simulink model "Robot"  (R2022b)
settings: Solver=FixedStepDiscrete  StartTime=0.0  StopTime=30  FixedStep=0.001  RelTol=1e-3
InitFcn:
  | load("BusConfig.mat");
undefined symbols (not defined in the file or in its folder): DiscIntNeverNeededParam
libraries: slrealtimeethercatlib x119, simulink x20
(part 4 of 7)

== system Robot/Motor4 Torque Control Init Frame/SDO Set 0x6040:6 Frame ==
  FinishIndex : Inport
  Enable : EnablePort
  Bitwise Operator : simulink/Logic and Bit Operations/Bitwise Operator  logicop=AND  UseBitMask=on  BitMask=bin2dec('0000000000000001')  BitMaskRealWorld=Stored Integer
  Clock : Clock
  Constant : Constant  Value=6  OutDataTypeStr=uint16
  Constant1 : Constant  OutDataTypeStr=int32
  Constant2 : Constant  Value=0  OutDataTypeStr=int32
  Constant4 : Constant  Value=0  OutDataTypeStr=double
  Constant5 : Constant
  Constant6 : Constant  OutDataTypeStr=int32
  Constant7 : Constant
  Constant8 : Constant  Value=0b0000000000000001  OutDataTypeStr=uint16
  Display{1..6} (6 alike) : Display
  EtherCAT Async SDO Download : slrealtimeethercatlib/EtherCAT Async SDO Download  index=0x6040  subIndex=0  sig_type=uint16  sig_dim=1  device_id=0  slave_name=Drive 4 (Elmo Drive )  sample_time=-1  slave_addr=1004  selected_slave=Term 1 (EK1100)  timeout=3000  slave_found=1  complete=0
  EtherCAT PDO Receive1 : slrealtimeethercatlib/EtherCAT PDO Receive  Priority=2  sig_name=Drive 4 (Elmo Drive ).Inputs.Status word  sig_offset=39136  sig_type=uint16  type_size=16  sig_dim=1  device_id=0  sample_time=0.001
  If Action Subsystem1 : Subsystem  TreatAsAtomicUnit=on
  If Action Subsystem2 : Subsystem  TreatAsAtomicUnit=on
  If Action Subsystem3 : Subsystem  TreatAsAtomicUnit=on
  If Action Subsystem5 : Subsystem  TreatAsAtomicUnit=on
  If Action Subsystem6 : Subsystem  TreatAsAtomicUnit=on
  If Action Subsystem7 : Subsystem  TreatAsAtomicUnit=on
  If1 : If  IfExpression=(u1 == 4663)
  If2 : If  IfExpression=(u1 == 2)
  If3 : If  NumInputs=2  IfExpression=(u1 == u2)
  If4 : If  IfExpression=(u1 >= 0.1)
  Merge1 : Merge
  Merge2 : Merge
  TaskFinished : Outport
  wires:
  Constant2/1 -> If Action Subsystem1/1(In1)
  Constant/1 -> EtherCAT Async SDO Download/1
  If1/1 -> If Action Subsystem7/Action
  Constant4/1 -> If Action Subsystem6/1(In1)
  If4/1 -> If Action Subsystem1/Action
  If Action Subsystem1/1(Out1) -> Merge2/1
  If2/2 -> If Action Subsystem6/Action
  Bitwise Operator/1 -> If3/1
  FinishIndex/1 -> If Action Subsystem5/1(In1)
  EtherCAT Async SDO Download/2 -> Display2/1
  EtherCAT Async SDO Download/1 -> If2/1, Display1/1
  If2/1 -> If Action Subsystem5/Action
  If4/2 -> If Action Subsystem2/Action
  Constant5/1 -> If Action Subsystem7/1(In1)
  If Action Subsystem2/1(Out1) -> Merge2/2
  Constant7/1 -> If Action Subsystem3/1(In1)
  If Action Subsystem3/1(Out1) -> Display6/1, If4/1
  If Action Subsystem5/1(Out1) -> Merge1/1
  Constant6/1 -> If Action Subsystem2/1(In1)
  If Action Subsystem6/1(Out1) -> Merge1/2
  Constant1/1 -> EtherCAT Async SDO Download/2
  If3/1 -> If Action Subsystem3/Action
  If Action Subsystem7/1(Out1) -> Display5/1
  Constant8/1 -> If3/2
  EtherCAT PDO Receive1/1 -> Display3/1, Bitwise Operator/1
  Clock/1 -> Display4/1
  Merge1/1 -> TaskFinished/1

== system Robot/Motor4 Torque Control Init Frame/SDO Set 0x6040:7 Frame ==
  FinishIndex : Inport
  Enable : EnablePort
  Bitwise Operator : simulink/Logic and Bit Operations/Bitwise Operator  logicop=AND  UseBitMask=on  BitMask=bin2dec('0000000000000011')  BitMaskRealWorld=Stored Integer
  Clock : Clock
  Constant : Constant  Value=7  OutDataTypeStr=uint16
  Constant1 : Constant  OutDataTypeStr=int32
  Constant2 : Constant  Value=0  OutDataTypeStr=int32
  Constant4 : Constant  Value=0  OutDataTypeStr=double
  Constant5 : Constant
  Constant6 : Constant  OutDataTypeStr=int32
  Constant7 : Constant
  Constant8 : Constant  Value=0b0000000000000011  OutDataTypeStr=uint16
  Display{1..6} (6 alike) : Display
  EtherCAT Async SDO Download : slrealtimeethercatlib/EtherCAT Async SDO Download  index=0x6040  subIndex=0  sig_type=uint16  sig_dim=1  device_id=0  slave_name=Drive 4 (Elmo Drive )  sample_time=-1  slave_addr=1004  selected_slave=Term 1 (EK1100)  timeout=2000  slave_found=1  complete=0
  EtherCAT PDO Receive1 : slrealtimeethercatlib/EtherCAT PDO Receive  Priority=2  sig_name=Drive 4 (Elmo Drive ).Inputs.Status word  sig_offset=39136  sig_type=uint16  type_size=16  sig_dim=1  device_id=0  sample_time=0.001
  If Action Subsystem1 : Subsystem  TreatAsAtomicUnit=on
  If Action Subsystem2 : Subsystem  TreatAsAtomicUnit=on
  If Action Subsystem3 : Subsystem  TreatAsAtomicUnit=on
  If Action Subsystem5 : Subsystem  TreatAsAtomicUnit=on
  If Action Subsystem6 : Subsystem  TreatAsAtomicUnit=on
  If Action Subsystem7 : Subsystem  TreatAsAtomicUnit=on
  If1 : If  IfExpression=(u1 == 4663)
  If2 : If  IfExpression=(u1 == 2)
  If3 : If  NumInputs=2  IfExpression=(u1 == u2)
  If4 : If  IfExpression=(u1 >= 0.1)
  Merge1 : Merge
  Merge2 : Merge
  TaskFinished : Outport
  wires:
  EtherCAT PDO Receive1/1 -> Display3/1, Bitwise Operator/1
  Constant1/1 -> EtherCAT Async SDO Download/2
  Constant/1 -> EtherCAT Async SDO Download/1
  If Action Subsystem1/1(Out1) -> Merge2/1
  Constant7/1 -> If Action Subsystem3/1(In1)
  EtherCAT Async SDO Download/2 -> Display2/1
  Constant4/1 -> If Action Subsystem6/1(In1)
  FinishIndex/1 -> If Action Subsystem5/1(In1)
  If Action Subsystem6/1(Out1) -> Merge1/2
  Constant2/1 -> If Action Subsystem1/1(In1)
  If Action Subsystem5/1(Out1) -> Merge1/1
  Constant5/1 -> If Action Subsystem7/1(In1)
  If4/2 -> If Action Subsystem2/Action
  If2/1 -> If Action Subsystem5/Action
  If Action Subsystem7/1(Out1) -> Display5/1
  Merge1/1 -> TaskFinished/1
  Constant6/1 -> If Action Subsystem2/1(In1)
  Bitwise Operator/1 -> If3/1
  If Action Subsystem3/1(Out1) -> Display6/1, If4/1
  If1/1 -> If Action Subsystem7/Action
  If4/1 -> If Action Subsystem1/Action
  Clock/1 -> Display4/1
  If3/1 -> If Action Subsystem3/Action
  If Action Subsystem2/1(Out1) -> Merge2/2
  Constant8/1 -> If3/2
  If2/2 -> If Action Subsystem6/Action
  EtherCAT Async SDO Download/1 -> If2/1, Display1/1

== system Robot/Motor4 Torque Control Init Frame/SDO Set 0x6060:10 Frame ==
  FinishIndex : Inport
  Enable : EnablePort
  Clock : Clock
  Constant : Constant  Value=10  OutDataTypeStr=int8
  Constant1 : Constant  OutDataTypeStr=int32
  Constant4 : Constant  Value=0  OutDataTypeStr=double
  Constant5 : Constant
  Display{1..2,4..5} (4 alike) : Display
  EtherCAT Async SDO Download : slrealtimeethercatlib/EtherCAT Async SDO Download  index=0x6060  subIndex=0  sig_type=int8  sig_dim=1  device_id=0  slave_name=Drive 4 (Elmo Drive )  sample_time=-1  slave_addr=1004  selected_slave=Term 1 (EK1100)  timeout=2000  slave_found=1  complete=0
  If Action Subsystem5 : Subsystem  TreatAsAtomicUnit=on
  If Action Subsystem6 : Subsystem  TreatAsAtomicUnit=on
  If Action Subsystem7 : Subsystem  TreatAsAtomicUnit=on
  If1 : If  IfExpression=(u1 == 4663)
  If2 : If  IfExpression=(u1 == 2)
  Merge1 : Merge
  TaskFinished : Outport
  wires:
  EtherCAT Async SDO Download/2 -> Display2/1
  If Action Subsystem7/1(Out1) -> Display5/1
  If Action Subsystem6/1(Out1) -> Merge1/2
  If2/1 -> If Action Subsystem5/Action
  If2/2 -> If Action Subsystem6/Action
  Constant/1 -> EtherCAT Async SDO Download/1
  If1/1 -> If Action Subsystem7/Action
  Merge1/1 -> TaskFinished/1
  If Action Subsystem5/1(Out1) -> Merge1/1
  Constant5/1 -> If Action Subsystem7/1(In1)
  Clock/1 -> Display4/1
  Constant1/1 -> EtherCAT Async SDO Download/2
  Constant4/1 -> If Action Subsystem6/1(In1)
  FinishIndex/1 -> If Action Subsystem5/1(In1)
  EtherCAT Async SDO Download/1 -> If2/1, Display1/1

== system Robot/Motor4 Torque Control Init Frame/SDO Set 0x6060:6 Frame ==
  FinishIndex : Inport
  Enable : EnablePort
  Clock : Clock
  Constant : Constant  Value=6  OutDataTypeStr=int8
  Constant1 : Constant  OutDataTypeStr=int32
  Constant4 : Constant  Value=0  OutDataTypeStr=double
  Constant5 : Constant
  Display{1..2,4..5} (4 alike) : Display
  EtherCAT Async SDO Download : slrealtimeethercatlib/EtherCAT Async SDO Download  index=0x6060  subIndex=0  sig_type=int8  sig_dim=1  device_id=0  slave_name=Drive 4 (Elmo Drive )  sample_time=-1  slave_addr=1004  selected_slave=Term 1 (EK1100)  timeout=2000  slave_found=1  complete=0
  If Action Subsystem5 : Subsystem  TreatAsAtomicUnit=on
  If Action Subsystem6 : Subsystem  TreatAsAtomicUnit=on
  If Action Subsystem7 : Subsystem  TreatAsAtomicUnit=on
  If1 : If  IfExpression=(u1 == 4663)
  If2 : If  IfExpression=(u1 == 2)
  Merge1 : Merge
  TaskFinished : Outport
  wires:
  FinishIndex/1 -> If Action Subsystem5/1(In1)
  If2/1 -> If Action Subsystem5/Action
  If Action Subsystem5/1(Out1) -> Merge1/1
  If Action Subsystem6/1(Out1) -> Merge1/2
  EtherCAT Async SDO Download/2 -> Display2/1
  If2/2 -> If Action Subsystem6/Action
  Constant1/1 -> EtherCAT Async SDO Download/2
  Merge1/1 -> TaskFinished/1
  If Action Subsystem7/1(Out1) -> Display5/1
  Clock/1 -> Display4/1
  EtherCAT Async SDO Download/1 -> If2/1, Display1/1
  Constant4/1 -> If Action Subsystem6/1(In1)
  Constant5/1 -> If Action Subsystem7/1(In1)
  If1/1 -> If Action Subsystem7/Action
  Constant/1 -> EtherCAT Async SDO Download/1

== system Robot/Motor4 Torque Control Init Frame/SDO Set 0x6080:-1 Frame ==
  FinishIndex : Inport
  Enable : EnablePort
  Clock : Clock
  Constant : Constant  Value=(2^31)-1  OutDataTypeStr=int32
  Constant1 : Constant  OutDataTypeStr=int32
  Constant4 : Constant  Value=0  OutDataTypeStr=double
  Constant5 : Constant
  Display{1..2,4..5} (4 alike) : Display
  EtherCAT Async SDO Download : slrealtimeethercatlib/EtherCAT Async SDO Download  index=0x6080  subIndex=0  sig_type=int32  sig_dim=1  device_id=0  slave_name=Drive 4 (Elmo Drive )  sample_time=-1  slave_addr=1004  selected_slave=Term 1 (EK1100)  timeout=3000  slave_found=1  complete=0
  If Action Subsystem5 : Subsystem  TreatAsAtomicUnit=on
  If Action Subsystem6 : Subsystem  TreatAsAtomicUnit=on
  If Action Subsystem7 : Subsystem  TreatAsAtomicUnit=on
  If1 : If  IfExpression=(u1 == 4663)
  If2 : If  IfExpression=(u1 == 2)
  Merge1 : Merge
  TaskFinished : Outport
  wires:
  Merge1/1 -> TaskFinished/1
  EtherCAT Async SDO Download/1 -> If2/1, Display1/1
  EtherCAT Async SDO Download/2 -> Display2/1
  Constant1/1 -> EtherCAT Async SDO Download/2
  FinishIndex/1 -> If Action Subsystem5/1(In1)
  If2/2 -> If Action Subsystem6/Action
  If2/1 -> If Action Subsystem5/Action
  Constant4/1 -> If Action Subsystem6/1(In1)
  Constant/1 -> EtherCAT Async SDO Download/1
  Constant5/1 -> If Action Subsystem7/1(In1)
  Clock/1 -> Display4/1
  If1/1 -> If Action Subsystem7/Action
  If Action Subsystem7/1(Out1) -> Display5/1
  If Action Subsystem6/1(Out1) -> Merge1/2
  If Action Subsystem5/1(Out1) -> Merge1/1

== system Robot/Motor4 Torque Control Init Frame/SDO Set 0x6098:35 Frame ==
  FinishIndex : Inport
  Enable : EnablePort
  Clock : Clock
  Constant : Constant  Value=35  OutDataTypeStr=int8
  Constant1 : Constant  OutDataTypeStr=int32
  Constant4 : Constant  Value=0  OutDataTypeStr=double
  Constant5 : Constant
  Display{1..2,4..5} (4 alike) : Display
  EtherCAT Async SDO Download : slrealtimeethercatlib/EtherCAT Async SDO Download  index=0x6098  subIndex=0  sig_type=int8  sig_dim=1  device_id=0  slave_name=Drive 4 (Elmo Drive )  sample_time=-1  slave_addr=1004  selected_slave=Term 1 (EK1100)  timeout=2000  slave_found=1  complete=0
  If Action Subsystem5 : Subsystem  TreatAsAtomicUnit=on
  If Action Subsystem6 : Subsystem  TreatAsAtomicUnit=on
  If Action Subsystem7 : Subsystem  TreatAsAtomicUnit=on
  If1 : If  IfExpression=(u1 == 4663)
  If2 : If  IfExpression=(u1 == 2)
  Merge1 : Merge
  TaskFinished : Outport
  wires:
  EtherCAT Async SDO Download/2 -> Display2/1
  EtherCAT Async SDO Download/1 -> If2/1, Display1/1
  Constant1/1 -> EtherCAT Async SDO Download/2
  FinishIndex/1 -> If Action Subsystem5/1(In1)
  Constant4/1 -> If Action Subsystem6/1(In1)
  If Action Subsystem5/1(Out1) -> Merge1/1
  Constant5/1 -> If Action Subsystem7/1(In1)
  Merge1/1 -> TaskFinished/1
  If2/1 -> If Action Subsystem5/Action
  If Action Subsystem7/1(Out1) -> Display5/1
  Constant/1 -> EtherCAT Async SDO Download/1
  If2/2 -> If Action Subsystem6/Action
  If Action Subsystem6/1(Out1) -> Merge1/2
  If1/1 -> If Action Subsystem7/Action
  Clock/1 -> Display4/1

== system Robot/Motor4 Torque Control Init Frame/Set MasterState to OP Frame ==
  FinishIndex : Inport
  Enable : EnablePort
  Clock : Clock
  Constant1 : Constant  OutDataTypeStr=boolean
  Constant2 : Constant  Value=8  OutDataTypeStr=int32
  Constant4 : Constant  Value=0  OutDataTypeStr=double
  Constant5 : Constant
  Display{1..2,4..5} (4 alike) : Display
  If Action Subsystem5 : Subsystem  TreatAsAtomicUnit=on
  If Action Subsystem6 : Subsystem  TreatAsAtomicUnit=on
  If Action Subsystem7 : Subsystem  TreatAsAtomicUnit=on
  If1 : If  IfExpression=(u1 == 8)
  If2 : If  IfExpression=(u1 > 0.1)
  Merge1 : Merge
  Set Device State : slrealtimeethercatlib/Set Device State  device_id=0  slave_name=Drive 4 (Elmo Drive )  sample_time=-1  slave_addr=1004  selected_slave=Term 1 (EK1100)  slave_found=1
  TaskFinished : Outport
  wires:
  Set Device State/1 -> If1/1, Display1/1
  Merge1/1 -> TaskFinished/1
  Constant1/1 -> Set Device State/2
  Constant4/1 -> If Action Subsystem6/1(In1)
  If1/1 -> If Action Subsystem7/Action
  FinishIndex/1 -> If Action Subsystem5/1(In1)
  Clock/1 -> Display4/1
  Set Device State/2 -> Display2/1
  If Action Subsystem5/1(Out1) -> Merge1/1
  If2/2 -> If Action Subsystem6/Action
  If2/1 -> If Action Subsystem5/Action
  If Action Subsystem7/1(Out1) -> If2/1, Display5/1
  If Action Subsystem6/1(Out1) -> Merge1/2
  Constant2/1 -> Set Device State/1
  Constant5/1 -> If Action Subsystem7/1(In1)

== system Robot/Motor4 Torque Control Init Frame/Set MasterState to SafeOP Frame ==
  FinishIndex : Inport
  Enable : EnablePort
  Clock : Clock
  Constant1 : Constant  OutDataTypeStr=boolean
  Constant2 : Constant  Value=4  OutDataTypeStr=int32
  Constant4 : Constant  Value=0  OutDataTypeStr=double
  Constant5 : Constant
  Display{1..2,4..5} (4 alike) : Display
  If Action Subsystem5 : Subsystem  TreatAsAtomicUnit=on
  If Action Subsystem6 : Subsystem  TreatAsAtomicUnit=on
  If Action Subsystem7 : Subsystem  TreatAsAtomicUnit=on
  If1 : If  IfExpression=(u1 == 4)
  If2 : If  IfExpression=(u1 > 0.1)
  Merge1 : Merge
  Set Device State : slrealtimeethercatlib/Set Device State  device_id=0  slave_name=Drive 4 (Elmo Drive )  sample_time=-1  slave_addr=1004  selected_slave=Term 1 (EK1100)  slave_found=1
  TaskFinished : Outport
  wires:
  Merge1/1 -> TaskFinished/1
  Set Device State/1 -> If1/1, Display1/1
  Constant1/1 -> Set Device State/2
  Constant2/1 -> Set Device State/1
  If Action Subsystem7/1(Out1) -> If2/1, Display5/1
  Constant5/1 -> If Action Subsystem7/1(In1)
  Clock/1 -> Display4/1
  If1/1 -> If Action Subsystem7/Action
  If2/1 -> If Action Subsystem5/Action
  If2/2 -> If Action Subsystem6/Action
  Set Device State/2 -> Display2/1
  If Action Subsystem6/1(Out1) -> Merge1/2
  Constant4/1 -> If Action Subsystem6/1(In1)
  FinishIndex/1 -> If Action Subsystem5/1(In1)
  If Action Subsystem5/1(Out1) -> Merge1/1

== system Robot/Motor4 Torque Control Init Frame/State_10_Enable ==
  State : Inport
  Subsystem : Subsystem
  Switch Case : SwitchCase  CaseConditions={TaskIndex}
  Enable : Outport
  FinishIndex : Outport  Port=2
  wires:
  Switch Case/2 -> Subsystem/2(Case Default)
  Switch Case/1 -> Subsystem/1(Case)
  Subsystem/2(FinishIndex) -> FinishIndex/1
  Subsystem/1(Enable) -> Enable/1
  State/1 -> Switch Case/1

== system Robot/Motor4 Torque Control Init Frame/State_11_Enable ==
  State : Inport
  Subsystem : Subsystem
  Switch Case : SwitchCase  CaseConditions={TaskIndex}
  Enable : Outport
  FinishIndex : Outport  Port=2
  wires:
  Switch Case/2 -> Subsystem/2(Case Default)
  Switch Case/1 -> Subsystem/1(Case)
  Subsystem/2(FinishIndex) -> FinishIndex/1
  Subsystem/1(Enable) -> Enable/1
  State/1 -> Switch Case/1

== system Robot/Motor4 Torque Control Init Frame/State_12_Enable ==
  State : Inport
  Subsystem : Subsystem
  Switch Case : SwitchCase  CaseConditions={TaskIndex}
  Enable : Outport
  FinishIndex : Outport  Port=2
  wires:
  Switch Case/2 -> Subsystem/2(Case Default)
  Switch Case/1 -> Subsystem/1(Case)
  Subsystem/2(FinishIndex) -> FinishIndex/1
  Subsystem/1(Enable) -> Enable/1
  State/1 -> Switch Case/1

== system Robot/Motor4 Torque Control Init Frame/State_13_Enable ==
  State : Inport
  Subsystem : Subsystem
  Switch Case : SwitchCase  CaseConditions={TaskIndex}
  Enable : Outport
  FinishIndex : Outport  Port=2
  wires:
  Switch Case/2 -> Subsystem/2(Case Default)
  Switch Case/1 -> Subsystem/1(Case)
  Subsystem/2(FinishIndex) -> FinishIndex/1
  Subsystem/1(Enable) -> Enable/1
  State/1 -> Switch Case/1

== system Robot/Motor4 Torque Control Init Frame/State_1_Enable ==
  State : Inport
  Subsystem : Subsystem
  Switch Case : SwitchCase  CaseConditions={TaskIndex}
  Enable : Outport
  FinishIndex : Outport  Port=2
  wires:
  Switch Case/2 -> Subsystem/2(Case Default)
  Switch Case/1 -> Subsystem/1(Case)
  Subsystem/2(FinishIndex) -> FinishIndex/1
  Subsystem/1(Enable) -> Enable/1
  State/1 -> Switch Case/1

== system Robot/Motor4 Torque Control Init Frame/State_2_Enable ==
  State : Inport
  Subsystem : Subsystem
  Switch Case : SwitchCase  CaseConditions={TaskIndex}
  Enable : Outport
  FinishIndex : Outport  Port=2
  wires:
  Switch Case/2 -> Subsystem/2(Case Default)
  Switch Case/1 -> Subsystem/1(Case)
  Subsystem/2(FinishIndex) -> FinishIndex/1
  Subsystem/1(Enable) -> Enable/1
  State/1 -> Switch Case/1

== system Robot/Motor4 Torque Control Init Frame/State_3_Enable ==
  State : Inport
  Subsystem : Subsystem
  Switch Case : SwitchCase  CaseConditions={TaskIndex}
  Enable : Outport
  FinishIndex : Outport  Port=2
  wires:
  Switch Case/2 -> Subsystem/2(Case Default)
  Switch Case/1 -> Subsystem/1(Case)
  Subsystem/2(FinishIndex) -> FinishIndex/1
  Subsystem/1(Enable) -> Enable/1
  State/1 -> Switch Case/1

== system Robot/Motor4 Torque Control Init Frame/State_4_Enable ==
  State : Inport
  Subsystem : Subsystem
  Switch Case : SwitchCase  CaseConditions={TaskIndex}
  Enable : Outport
  FinishIndex : Outport  Port=2
  wires:
  Switch Case/2 -> Subsystem/2(Case Default)
  Switch Case/1 -> Subsystem/1(Case)
  Subsystem/2(FinishIndex) -> FinishIndex/1
  Subsystem/1(Enable) -> Enable/1
  State/1 -> Switch Case/1

== system Robot/Motor4 Torque Control Init Frame/State_5_Enable ==
  State : Inport
  Subsystem : Subsystem
  Switch Case : SwitchCase  CaseConditions={TaskIndex}
  Enable : Outport
  FinishIndex : Outport  Port=2
  wires:
  Switch Case/2 -> Subsystem/2(Case Default)
  Switch Case/1 -> Subsystem/1(Case)
  Subsystem/2(FinishIndex) -> FinishIndex/1
  Subsystem/1(Enable) -> Enable/1
  State/1 -> Switch Case/1

== system Robot/Motor4 Torque Control Init Frame/State_6_Enable ==
  State : Inport
  Subsystem : Subsystem
  Switch Case : SwitchCase  CaseConditions={TaskIndex}
  Enable : Outport
  FinishIndex : Outport  Port=2
  wires:
  Switch Case/2 -> Subsystem/2(Case Default)
  Switch Case/1 -> Subsystem/1(Case)
  Subsystem/2(FinishIndex) -> FinishIndex/1
  Subsystem/1(Enable) -> Enable/1
  State/1 -> Switch Case/1

== system Robot/Motor4 Torque Control Init Frame/State_7_Enable ==
  State : Inport
  Subsystem : Subsystem
  Switch Case : SwitchCase  CaseConditions={TaskIndex}
  Enable : Outport
  FinishIndex : Outport  Port=2
  wires:
  Switch Case/2 -> Subsystem/2(Case Default)
  Switch Case/1 -> Subsystem/1(Case)
  Subsystem/2(FinishIndex) -> FinishIndex/1
  Subsystem/1(Enable) -> Enable/1
  State/1 -> Switch Case/1

== system Robot/Motor4 Torque Control Init Frame/State_8_Enable ==
  State : Inport
  Subsystem : Subsystem
  Switch Case : SwitchCase  CaseConditions={TaskIndex}
  Enable : Outport
  FinishIndex : Outport  Port=2
  wires:
  Switch Case/2 -> Subsystem/2(Case Default)
  Switch Case/1 -> Subsystem/1(Case)
  Subsystem/2(FinishIndex) -> FinishIndex/1
  Subsystem/1(Enable) -> Enable/1
  State/1 -> Switch Case/1

== system Robot/Motor4 Torque Control Init Frame/State_9_Enable ==
  State : Inport
  Subsystem : Subsystem
  Switch Case : SwitchCase  CaseConditions={TaskIndex}
  Enable : Outport
  FinishIndex : Outport  Port=2
  wires:
  Switch Case/2 -> Subsystem/2(Case Default)
  Switch Case/1 -> Subsystem/1(Case)
  Subsystem/2(FinishIndex) -> FinishIndex/1
  Subsystem/1(Enable) -> Enable/1
  State/1 -> Switch Case/1

== system Robot/State_1_Enable/Subsystem ==
  Case : Inport
  Case Default : Inport  Port=2
  Constant : Constant
  Constant1 : Constant  Value=0
  Constant2 : Constant  Value=TaskIndex
  Merge : Merge
  Switch Case Action Subsystem : Subsystem  TreatAsAtomicUnit=on
  Switch Case Action Subsystem1 : Subsystem  TreatAsAtomicUnit=on
  Enable : Outport
  FinishIndex : Outport  Port=2
  wires:
  Constant/1 -> Switch Case Action Subsystem/1(In1)
  Case/1 -> Switch Case Action Subsystem/Action
  Switch Case Action Subsystem/1(Out1) -> Merge/1
  Merge/1 -> Enable/1
  Case Default/1 -> Switch Case Action Subsystem1/Action
  Constant1/1 -> Switch Case Action Subsystem1/1(In1)
  Switch Case Action Subsystem1/1(Default) -> Merge/2
  Constant2/1 -> FinishIndex/1

== system Robot/State_2_Enable/Subsystem ==
  Case : Inport
  Case Default : Inport  Port=2
  Constant : Constant
  Constant1 : Constant  Value=0
  Constant2 : Constant  Value=TaskIndex
  Merge : Merge
  Switch Case Action Subsystem : Subsystem  TreatAsAtomicUnit=on
  Switch Case Action Subsystem1 : Subsystem  TreatAsAtomicUnit=on
  Enable : Outport
  FinishIndex : Outport  Port=2
  wires:
  Constant/1 -> Switch Case Action Subsystem/1(In1)
  Case/1 -> Switch Case Action Subsystem/Action
  Switch Case Action Subsystem/1(Out1) -> Merge/1
  Merge/1 -> Enable/1
  Case Default/1 -> Switch Case Action Subsystem1/Action
  Constant1/1 -> Switch Case Action Subsystem1/1(In1)
  Switch Case Action Subsystem1/1(Default) -> Merge/2
  Constant2/1 -> FinishIndex/1

== system Robot/State_3_Enable/Subsystem ==
  Case : Inport
  Case Default : Inport  Port=2
  Constant : Constant
  Constant1 : Constant  Value=0
  Constant2 : Constant  Value=TaskIndex
  Merge : Merge
  Switch Case Action Subsystem : Subsystem  TreatAsAtomicUnit=on
  Switch Case Action Subsystem1 : Subsystem  TreatAsAtomicUnit=on
  Enable : Outport
  FinishIndex : Outport  Port=2
  wires:
  Constant/1 -> Switch Case Action Subsystem/1(In1)
  Case/1 -> Switch Case Action Subsystem/Action
  Switch Case Action Subsystem/1(Out1) -> Merge/1
  Merge/1 -> Enable/1
  Case Default/1 -> Switch Case Action Subsystem1/Action
  Constant1/1 -> Switch Case Action Subsystem1/1(In1)
  Switch Case Action Subsystem1/1(Default) -> Merge/2
  Constant2/1 -> FinishIndex/1

== system Robot/State_4_Enable/Subsystem ==
  Case : Inport
  Case Default : Inport  Port=2
  Constant : Constant
  Constant1 : Constant  Value=0
  Constant2 : Constant  Value=TaskIndex
  Merge : Merge
  Switch Case Action Subsystem : Subsystem  TreatAsAtomicUnit=on
  Switch Case Action Subsystem1 : Subsystem  TreatAsAtomicUnit=on
  Enable : Outport
  FinishIndex : Outport  Port=2
  wires:
  Constant/1 -> Switch Case Action Subsystem/1(In1)
  Case/1 -> Switch Case Action Subsystem/Action
  Switch Case Action Subsystem/1(Out1) -> Merge/1
  Merge/1 -> Enable/1
  Case Default/1 -> Switch Case Action Subsystem1/Action
  Constant1/1 -> Switch Case Action Subsystem1/1(In1)
  Switch Case Action Subsystem1/1(Default) -> Merge/2
  Constant2/1 -> FinishIndex/1

== system Robot/State_5_Enable/Subsystem ==
  Case : Inport
  Case Default : Inport  Port=2
  Constant : Constant
  Constant1 : Constant  Value=0
  Constant2 : Constant  Value=TaskIndex
  Merge : Merge
  Switch Case Action Subsystem : Subsystem  TreatAsAtomicUnit=on
  Switch Case Action Subsystem1 : Subsystem  TreatAsAtomicUnit=on
  Enable : Outport
  FinishIndex : Outport  Port=2
  wires:
  Constant/1 -> Switch Case Action Subsystem/1(In1)
  Case/1 -> Switch Case Action Subsystem/Action
  Switch Case Action Subsystem/1(Out1) -> Merge/1
  Merge/1 -> Enable/1
  Case Default/1 -> Switch Case Action Subsystem1/Action
  Constant1/1 -> Switch Case Action Subsystem1/1(In1)
  Switch Case Action Subsystem1/1(Default) -> Merge/2
  Constant2/1 -> FinishIndex/1

== system Robot/Subsystem/M1_Current->TorqueCommand ==
  Current : Inport
  RatedCurrent : Inport  Port=2
  Data Type Conversion1 : DataTypeConversion  OutDataTypeStr=int16  SaturateOnIntegerOverflow=off  RndMeth=Floor
  Display1 : Display
  Divide2 : Product  Inputs=*/
  Gain1 : Gain  Gain=1000*1000
  Command : Outport
  wires:
  RatedCurrent/1 -> Divide2/2
  Gain1/1 -> Divide2/1
  Divide2/1 -> Display1/1, Data Type Conversion1/1
  Current/1 -> Gain1/1
  Data Type Conversion1/1 -> Command/1

== system Robot/Subsystem/M24_Current->TorqueCommand ==
  Current : Inport
  RatedCurrent : Inport  Port=2
  Data Type Conversion1 : DataTypeConversion  OutDataTypeStr=int16  SaturateOnIntegerOverflow=off  RndMeth=Floor
  Display1 : Display
  Divide2 : Product  Inputs=*/
  Gain1 : Gain  Gain=1000*1000
  Command : Outport
  wires:
  RatedCurrent/1 -> Divide2/2
  Gain1/1 -> Divide2/1
  Divide2/1 -> Display1/1, Data Type Conversion1/1
  Current/1 -> Gain1/1
  Data Type Conversion1/1 -> Command/1

== system Robot/Subsystem/M2_Current->TorqueCommand ==
  Current : Inport
  RatedCurrent : Inport  Port=2
  Data Type Conversion1 : DataTypeConversion  OutDataTypeStr=int16  SaturateOnIntegerOverflow=off  RndMeth=Floor
  Display1 : Display
  Divide2 : Product  Inputs=*/
  Gain1 : Gain  Gain=1000*1000
  Command : Outport
  wires:
  RatedCurrent/1 -> Divide2/2
  Gain1/1 -> Divide2/1
  Divide2/1 -> Display1/1, Data Type Conversion1/1
  Current/1 -> Gain1/1
  Data Type Conversion1/1 -> Command/1

== system Robot/Subsystem/M3_Cnt->Deg ==
  note: Unit:Degree/Second
  M3_ActuralVelocity : Inport
  Data Type Conversion7 : DataTypeConversion  OutDataTypeStr=double  SaturateOnIntegerOverflow=off  RndMeth=Floor
  Gain6 : Gain  Gain=360/(8192*9*2)
  Motor1ActuralVelocity : Outport
  wires:
  Gain6/1 -> Data Type Conversion7/1
  M3_ActuralVelocity/1 -> Gain6/1
  Data Type Conversion7/1 -> Motor1ActuralVelocity/1

== system Robot/Subsystem/M3_Command->Current ==
  note: Unit:A
  RatedCurrent : Inport
  Command : Inport  Port=2
  Data Type Conversion2 : DataTypeConversion  OutDataTypeStr=int16  SaturateOnIntegerOverflow=off  RndMeth=Floor
  Data Type Conversion4 : DataTypeConversion  OutDataTypeStr=double  SaturateOnIntegerOverflow=off  RndMeth=Floor
  Dot Product : DotProduct  OutDataTypeStr=Inherit: Inherit via internal rule
  Gain2 : Gain  Gain=1/(1000*1000)
  Current : Outport
  wires:
  Gain2/1 -> Data Type Conversion4/1
  RatedCurrent/1 -> Data Type Conversion2/1
  Dot Product/1 -> Gain2/1
  Command/1 -> Dot Product/2
  Data Type Conversion2/1 -> Dot Product/1
  Data Type Conversion4/1 -> Current/1

== system Robot/Subsystem/M3_Current->TorqueCommand ==
  Current : Inport
  RatedCurrent : Inport  Port=2
  Data Type Conversion1 : DataTypeConversion  OutDataTypeStr=int16  SaturateOnIntegerOverflow=off  RndMeth=Floor
  Display1 : Display
  Divide2 : Product  Inputs=*/
  Gain1 : Gain  Gain=1000*1000
  Command : Outport
  wires:
  RatedCurrent/1 -> Divide2/2
  Gain1/1 -> Divide2/1
  Divide2/1 -> Display1/1, Data Type Conversion1/1
  Current/1 -> Gain1/1
  Data Type Conversion1/1 -> Command/1

== system Robot/Subsystem/M3_PositionCalibrate ==
  note: Unit:Degree
  M3_ActuralPosition : Inport
  Bias : Bias  Commented=through  Bias=-43  SaturateOnIntegerOverflow=off
  Bias2 : Bias  Bias=-3388710  SaturateOnIntegerOverflow=off
  Data Type Conversion6 : DataTypeConversion  OutDataTypeStr=double  SaturateOnIntegerOverflow=off  RndMeth=Floor
  Gain4 : Gain  Gain=360/(8192*9*2)
  Motor1ActuralPosition : Outport
  wires:
  Gain4/1 -> Bias/1
  Bias2/1 -> Gain4/1
  Data Type Conversion6/1 -> Motor1ActuralPosition/1
  Bias/1 -> Data Type Conversion6/1
  M3_ActuralPosition/1 -> Bias2/1

== system Robot/Subsystem/M4_Cnt->Deg ==
  note: Unit:Degree/Second
  M3_ActuralVelocity : Inport
  Data Type Conversion7 : DataTypeConversion  OutDataTypeStr=double  SaturateOnIntegerOverflow=off  RndMeth=Floor
  Gain6 : Gain  Gain=360/(8192*9*2)
  Motor1ActuralVelocity : Outport
  wires:
  Gain6/1 -> Data Type Conversion7/1
  M3_ActuralVelocity/1 -> Gain6/1
  Data Type Conversion7/1 -> Motor1ActuralVelocity/1

== system Robot/Subsystem/M4_Command->Current ==
  note: Unit:A
  RatedCurrent : Inport
  Command : Inport  Port=2
  Data Type Conversion3 : DataTypeConversion  OutDataTypeStr=int16  SaturateOnIntegerOverflow=off  RndMeth=Floor
  Data Type Conversion5 : DataTypeConversion  OutDataTypeStr=double  SaturateOnIntegerOverflow=off  RndMeth=Floor
  Dot Product1 : DotProduct  OutDataTypeStr=Inherit: Inherit via internal rule
  Gain3 : Gain  Gain=1/(1000*1000)
  Current : Outport
  wires:
  Command/1 -> Dot Product1/2
  RatedCurrent/1 -> Data Type Conversion3/1
  Gain3/1 -> Data Type Conversion5/1
  Dot Product1/1 -> Gain3/1
  Data Type Conversion5/1 -> Current/1
  Data Type Conversion3/1 -> Dot Product1/1

== system Robot/Subsystem/M4_PositionCalibrate ==
  note: Unit:Degree
  M4_ActuralPosition : Inport
  Bias1 : Bias  Commented=through  Bias=-25  SaturateOnIntegerOverflow=off
  Bias3 : Bias  Bias=-9789179  SaturateOnIntegerOverflow=off
  Data Type Conversion9 : DataTypeConversion  OutDataTypeStr=double  SaturateOnIntegerOverflow=off  RndMeth=Floor
  Gain5 : Gain  Gain=360/(8192*9*2)
  Motor2ActuralPosition : Outport
  wires:
  Gain5/1 -> Bias1/1
  Bias3/1 -> Gain5/1
  Bias1/1 -> Data Type Conversion9/1
  M4_ActuralPosition/1 -> Bias3/1
  Data Type Conversion9/1 -> Motor2ActuralPosition/1

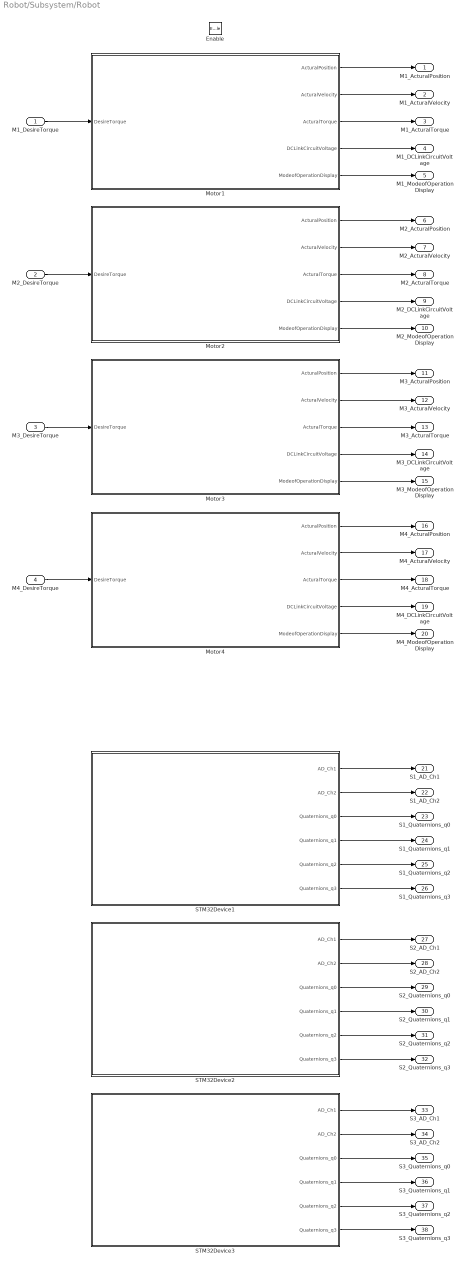
== system Robot/Subsystem/Robot ==
  M1_DesireTorque : Inport
  M2_DesireTorque : Inport  Port=2
  M3_DesireTorque : Inport  Port=3
  M4_DesireTorque : Inport  Port=4
  Enable : EnablePort
  Motor1 : Subsystem
  Motor2 : Subsystem
  Motor3 : Subsystem
  Motor4 : Subsystem
  STM32Device1 : Subsystem
  STM32Device2 : Subsystem
  STM32Device3 : Subsystem
  M1_ActuralPosition : Outport
  M1_ActuralVelocity : Outport  Port=2
  M1_ActuralTorque : Outport  Port=3
  M1_DCLinkCircuitVoltage : Outport  Port=4
  M1_ModeofOperationDisplay : Outport  Port=5
  M2_ActuralPosition : Outport  Port=6
  M2_ActuralVelocity : Outport  Port=7
  M2_ActuralTorque : Outport  Port=8
  M2_DCLinkCircuitVoltage : Outport  Port=9
  M2_ModeofOperationDisplay : Outport  Port=10
  M3_ActuralPosition : Outport  Port=11
  M3_ActuralVelocity : Outport  Port=12
  M3_ActuralTorque : Outport  Port=13
  M3_DCLinkCircuitVoltage : Outport  Port=14
  M3_ModeofOperationDisplay : Outport  Port=15
  M4_ActuralPosition : Outport  Port=16
  M4_ActuralVelocity : Outport  Port=17
  M4_ActuralTorque : Outport  Port=18
  M4_DCLinkCircuitVoltage : Outport  Port=19
  M4_ModeofOperationDisplay : Outport  Port=20
  S1_AD_Ch1 : Outport  Port=21
  S1_AD_Ch2 : Outport  Port=22
  S1_Quaternions_q0 : Outport  Port=23
  S1_Quaternions_q1 : Outport  Port=24
  S1_Quaternions_q2 : Outport  Port=25
  S1_Quaternions_q3 : Outport  Port=26
  S2_AD_Ch1 : Outport  Port=27
  S2_AD_Ch2 : Outport  Port=28
  S2_Quaternions_q0 : Outport  Port=29
  S2_Quaternions_q1 : Outport  Port=30
  S2_Quaternions_q2 : Outport  Port=31
  S2_Quaternions_q3 : Outport  Port=32
  S3_AD_Ch1 : Outport  Port=33
  S3_AD_Ch2 : Outport  Port=34
  S3_Quaternions_q0 : Outport  Port=35
  S3_Quaternions_q1 : Outport  Port=36
  S3_Quaternions_q2 : Outport  Port=37
  S3_Quaternions_q3 : Outport  Port=38
  wires:
  Motor1/5(ModeofOperationDisplay) -> M1_ModeofOperationDisplay/1
  Motor2/5(ModeofOperationDisplay) -> M2_ModeofOperationDisplay/1
  Motor1/3(ActuralTorque) -> M1_ActuralTorque/1
  STM32Device1/1(AD_Ch1) -> S1_AD_Ch1/1
  M2_DesireTorque/1 -> Motor2/1(DesireTorque)
  M1_DesireTorque/1 -> Motor1/1(DesireTorque)
  Motor2/4(DCLinkCircuitVoltage) -> M2_DCLinkCircuitVoltage/1
  STM32Device2/6(Quaternions_q3) -> S2_Quaternions_q3/1
  STM32Device3/5(Quaternions_q2) -> S3_Quaternions_q2/1
  Motor2/1(ActuralPosition) -> M2_ActuralPosition/1
  Motor1/2(ActuralVelocity) -> M1_ActuralVelocity/1
  Motor1/4(DCLinkCircuitVoltage) -> M1_DCLinkCircuitVoltage/1
  Motor1/1(ActuralPosition) -> M1_ActuralPosition/1
  Motor2/2(ActuralVelocity) -> M2_ActuralVelocity/1
  STM32Device2/4(Quaternions_q1) -> S2_Quaternions_q1/1
  STM32Device3/6(Quaternions_q3) -> S3_Quaternions_q3/1
  Motor2/3(ActuralTorque) -> M2_ActuralTorque/1
  STM32Device1/3(Quaternions_q0) -> S1_Quaternions_q0/1
  STM32Device3/1(AD_Ch1) -> S3_AD_Ch1/1
  STM32Device1/2(AD_Ch2) -> S1_AD_Ch2/1
  STM32Device1/4(Quaternions_q1) -> S1_Quaternions_q1/1
  STM32Device3/4(Quaternions_q1) -> S3_Quaternions_q1/1
  STM32Device2/1(AD_Ch1) -> S2_AD_Ch1/1
  STM32Device3/2(AD_Ch2) -> S3_AD_Ch2/1
  STM32Device1/6(Quaternions_q3) -> S1_Quaternions_q3/1
  STM32Device3/3(Quaternions_q0) -> S3_Quaternions_q0/1
  STM32Device1/5(Quaternions_q2) -> S1_Quaternions_q2/1
  STM32Device2/2(AD_Ch2) -> S2_AD_Ch2/1
  STM32Device2/5(Quaternions_q2) -> S2_Quaternions_q2/1
  STM32Device2/3(Quaternions_q0) -> S2_Quaternions_q0/1
  Motor3/4(DCLinkCircuitVoltage) -> M3_DCLinkCircuitVoltage/1
  Motor3/5(ModeofOperationDisplay) -> M3_ModeofOperationDisplay/1
  Motor3/3(ActuralTorque) -> M3_ActuralTorque/1
  Motor3/2(ActuralVelocity) -> M3_ActuralVelocity/1
  Motor3/1(ActuralPosition) -> M3_ActuralPosition/1
  Motor4/4(DCLinkCircuitVoltage) -> M4_DCLinkCircuitVoltage/1
  Motor4/5(ModeofOperationDisplay) -> M4_ModeofOperationDisplay/1
  Motor4/3(ActuralTorque) -> M4_ActuralTorque/1
  Motor4/2(ActuralVelocity) -> M4_ActuralVelocity/1
  Motor4/1(ActuralPosition) -> M4_ActuralPosition/1
  M3_DesireTorque/1 -> Motor3/1(DesireTorque)
  M4_DesireTorque/1 -> Motor4/1(DesireTorque)

== system Robot/Subsystem/S1ch1_ForceCalibrate ==
  In : Inport
  Bias : Bias  Bias=48  SaturateOnIntegerOverflow=off
  Data Type Conversion12 : DataTypeConversion  OutDataTypeStr=double  SaturateOnIntegerOverflow=off  RndMeth=Floor
  Gain8 : Gain  Gain=1.054*9.8*100*1000/(2.6363*5*1)
  Out : Outport
  wires:
  Bias/1 -> Data Type Conversion12/1
  In/1 -> Gain8/1
  Gain8/1 -> Bias/1
  Data Type Conversion12/1 -> Out/1

== system Robot/Subsystem/S1ch2_ForceCalibrate ==
  In : Inport
  Bias : Bias  Bias=44  SaturateOnIntegerOverflow=off
  Data Type Conversion12 : DataTypeConversion  OutDataTypeStr=double  SaturateOnIntegerOverflow=off  RndMeth=Floor
  Gain8 : Gain  Gain=1.093*9.8*100*1000/(2.6303*5*1)
  Out : Outport
  wires:
  Bias/1 -> Data Type Conversion12/1
  In/1 -> Gain8/1
  Gain8/1 -> Bias/1
  Data Type Conversion12/1 -> Out/1

== system Robot/Subsystem/S3ch1_ForceCalibrate ==
  In : Inport
  Bias : Bias  Bias=10  SaturateOnIntegerOverflow=off
  Data Type Conversion12 : DataTypeConversion  OutDataTypeStr=double  SaturateOnIntegerOverflow=off  RndMeth=Floor
  Gain8 : Gain  Gain=9.8*100*1000/(2.6185*5*1)
  Out : Outport
  wires:
  Bias/1 -> Data Type Conversion12/1
  In/1 -> Gain8/1
  Gain8/1 -> Bias/1
  Data Type Conversion12/1 -> Out/1

== system Robot/Subsystem/S3ch2_ForceCalibrate ==
  In : Inport
  Bias : Bias  Bias=10  SaturateOnIntegerOverflow=off
  Data Type Conversion12 : DataTypeConversion  OutDataTypeStr=double  SaturateOnIntegerOverflow=off  RndMeth=Floor
  Gain8 : Gain  Gain=9.8*100*1000/(2.6034*5*1)
  Out : Outport
  wires:
  Bias/1 -> Data Type Conversion12/1
  In/1 -> Gain8/1
  Gain8/1 -> Bias/1
  Data Type Conversion12/1 -> Out/1

== system Robot/Motor1 Torque Control Init Frame/Get MasterState OP Frame/If Action Subsystem5 ==
  In1 : Inport
  Action Port : ActionPort  ActionPortLabel=if((u1 == 8))
  Out1 : Outport
  wires:
  In1/1 -> Out1/1

== system Robot/Motor1 Torque Control Init Frame/Get MasterState OP Frame/If Action Subsystem6 ==
  In1 : Inport
  Action Port : ActionPort  ActionPortLabel=else
  Out1 : Outport
  wires:
  In1/1 -> Out1/1

== system Robot/Motor1 Torque Control Init Frame/Get MasterState OP Frame/If Action Subsystem7 ==
  In1 : Inport
  Action Port : ActionPort  ActionPortLabel=if((u1 == 4663))
  Discrete-Time Integrator : DiscreteIntegrator  SampleTime=-1  ICPrevOutput=DiscIntNeverNeededParam  ICPrevScaledInput=DiscIntNeverNeededParam
  Out1 : Outport
  wires:
  In1/1 -> Discrete-Time Integrator/1
  Discrete-Time Integrator/1 -> Out1/1

== system Robot/Motor1 Torque Control Init Frame/PDO Set 0x6040:6->7->15 Frame/If Action Subsystem ==
  In1 : Inport
  Action Port : ActionPort  ActionPortLabel=if((u1 == 720)&(u2 == 500))
  Out1 : Outport
  wires:
  In1/1 -> Out1/1

== system Robot/Motor1 Torque Control Init Frame/PDO Set 0x6040:6->7->15 Frame/If Action Subsystem1 ==
  In1 : Inport
  Action Port : ActionPort  ActionPortLabel=elseif((u1 == 689)&(u2 == 500))
  Out1 : Outport
  wires:
  In1/1 -> Out1/1

== system Robot/Motor1 Torque Control Init Frame/PDO Set 0x6040:6->7->15 Frame/If Action Subsystem2 ==
  In1 : Inport
  Action Port : ActionPort  ActionPortLabel=elseif( (u1 == 691)&(u2 == 500))
  Out1 : Outport
  wires:
  In1/1 -> Out1/1

== system Robot/Motor1 Torque Control Init Frame/PDO Set 0x6040:6->7->15 Frame/If Action Subsystem4 ==
  In1 : Inport
  Action Port : ActionPort  ActionPortLabel=else
  Out1 : Outport
  wires:
  In1/1 -> Out1/1

== system Robot/Motor1 Torque Control Init Frame/PDO Set 0x6040:6->7->15 Frame/If Action Subsystem5 ==
  In1 : Inport
  Action Port : ActionPort  ActionPortLabel=if((u1 >= 0.1))
  Out1 : Outport
  wires:
  In1/1 -> Out1/1

== system Robot/Motor1 Torque Control Init Frame/PDO Set 0x6040:6->7->15 Frame/If Action Subsystem6 ==
  In1 : Inport
  Action Port : ActionPort  ActionPortLabel=else
  Out1 : Outport
  wires:
  In1/1 -> Out1/1

== system Robot/Motor1 Torque Control Init Frame/PDO Set 0x6040:6->7->15 Frame/If Action Subsystem7 ==
  In1 : Inport
  Action Port : ActionPort  ActionPortLabel=if((u1 == 4663)|(u1 == 4791))
  Discrete-Time Integrator : DiscreteIntegrator  SampleTime=-1  ICPrevOutput=DiscIntNeverNeededParam  ICPrevScaledInput=DiscIntNeverNeededParam
  Out1 : Outport
  wires:
  In1/1 -> Discrete-Time Integrator/1
  Discrete-Time Integrator/1 -> Out1/1

== system Robot/Motor1 Torque Control Init Frame/SDO Get 0x6075 Frame/If Action Subsystem5 ==
  In1 : Inport
  Action Port : ActionPort  ActionPortLabel=if((u1 == 2))
  Out1 : Outport
  wires:
  In1/1 -> Out1/1

== system Robot/Motor1 Torque Control Init Frame/SDO Get 0x6075 Frame/If Action Subsystem6 ==
  In1 : Inport
  Action Port : ActionPort  ActionPortLabel=else
  Out1 : Outport
  wires:
  In1/1 -> Out1/1

== system Robot/Motor1 Torque Control Init Frame/SDO Get 0x6075 Frame/If Action Subsystem7 ==
  In1 : Inport
  Action Port : ActionPort  ActionPortLabel=if((u1 == 4663))
  Discrete-Time Integrator : DiscreteIntegrator  SampleTime=-1  ICPrevOutput=DiscIntNeverNeededParam  ICPrevScaledInput=DiscIntNeverNeededParam
  Out1 : Outport
  wires:
  In1/1 -> Discrete-Time Integrator/1
  Discrete-Time Integrator/1 -> Out1/1

== system Robot/Motor1 Torque Control Init Frame/SDO Set 0x6040:15 Frame/If Action Subsystem1 ==
  In1 : Inport
  Action Port : ActionPort  ActionPortLabel=if((u1 >= 0.1))
  Out1 : Outport
  wires:
  In1/1 -> Out1/1

== system Robot/Motor1 Torque Control Init Frame/SDO Set 0x6040:15 Frame/If Action Subsystem2 ==
  In1 : Inport
  Action Port : ActionPort  ActionPortLabel=else
  Out1 : Outport
  wires:
  In1/1 -> Out1/1

== system Robot/Motor1 Torque Control Init Frame/SDO Set 0x6040:15 Frame/If Action Subsystem3 ==
  In1 : Inport
  Action Port : ActionPort  ActionPortLabel=if((u1 == u2))
  Discrete-Time Integrator : DiscreteIntegrator  SampleTime=-1  ICPrevOutput=DiscIntNeverNeededParam  ICPrevScaledInput=DiscIntNeverNeededParam
  Out1 : Outport
  wires:
  In1/1 -> Discrete-Time Integrator/1
  Discrete-Time Integrator/1 -> Out1/1

== system Robot/Motor1 Torque Control Init Frame/SDO Set 0x6040:15 Frame/If Action Subsystem5 ==
  In1 : Inport
  Action Port : ActionPort  ActionPortLabel=if((u1 == 2))
  Out1 : Outport
  wires:
  In1/1 -> Out1/1

== system Robot/Motor1 Torque Control Init Frame/SDO Set 0x6040:15 Frame/If Action Subsystem6 ==
  In1 : Inport
  Action Port : ActionPort  ActionPortLabel=else
  Out1 : Outport
  wires:
  In1/1 -> Out1/1

== system Robot/Motor1 Torque Control Init Frame/SDO Set 0x6040:15 Frame/If Action Subsystem7 ==
  In1 : Inport
  Action Port : ActionPort  ActionPortLabel=if((u1 == 4663))
  Discrete-Time Integrator : DiscreteIntegrator  SampleTime=-1  ICPrevOutput=DiscIntNeverNeededParam  ICPrevScaledInput=DiscIntNeverNeededParam
  Out1 : Outport
  wires:
  In1/1 -> Discrete-Time Integrator/1
  Discrete-Time Integrator/1 -> Out1/1

== system Robot/Motor1 Torque Control Init Frame/SDO Set 0x6040:31 Frame/If Action Subsystem1 ==
  In1 : Inport
  Action Port : ActionPort  ActionPortLabel=if((u1 >= 0.1))
  Out1 : Outport
  wires:
  In1/1 -> Out1/1

== system Robot/Motor1 Torque Control Init Frame/SDO Set 0x6040:31 Frame/If Action Subsystem2 ==
  In1 : Inport
  Action Port : ActionPort  ActionPortLabel=else
  Out1 : Outport
  wires:
  In1/1 -> Out1/1

== system Robot/Motor1 Torque Control Init Frame/SDO Set 0x6040:31 Frame/If Action Subsystem3 ==
  In1 : Inport
  Action Port : ActionPort  ActionPortLabel=if((u1 == u2))
  Discrete-Time Integrator : DiscreteIntegrator  SampleTime=-1  ICPrevOutput=DiscIntNeverNeededParam  ICPrevScaledInput=DiscIntNeverNeededParam
  Out1 : Outport
  wires:
  In1/1 -> Discrete-Time Integrator/1
  Discrete-Time Integrator/1 -> Out1/1

== system Robot/Motor1 Torque Control Init Frame/SDO Set 0x6040:31 Frame/If Action Subsystem5 ==
  In1 : Inport
  Action Port : ActionPort  ActionPortLabel=if((u1 == 2))
  Out1 : Outport
  wires:
  In1/1 -> Out1/1

== system Robot/Motor1 Torque Control Init Frame/SDO Set 0x6040:31 Frame/If Action Subsystem6 ==
  In1 : Inport
  Action Port : ActionPort  ActionPortLabel=else
  Out1 : Outport
  wires:
  In1/1 -> Out1/1

== system Robot/Motor1 Torque Control Init Frame/SDO Set 0x6040:31 Frame/If Action Subsystem7 ==
  In1 : Inport
  Action Port : ActionPort  ActionPortLabel=if((u1 == 4663))
  Discrete-Time Integrator : DiscreteIntegrator  SampleTime=-1  ICPrevOutput=DiscIntNeverNeededParam  ICPrevScaledInput=DiscIntNeverNeededParam
  Out1 : Outport
  wires:
  In1/1 -> Discrete-Time Integrator/1
  Discrete-Time Integrator/1 -> Out1/1

== system Robot/Motor1 Torque Control Init Frame/SDO Set 0x6040:6 Frame/If Action Subsystem1 ==
  In1 : Inport
  Action Port : ActionPort  ActionPortLabel=if((u1 >= 0.1))
  Out1 : Outport
  wires:
  In1/1 -> Out1/1

== system Robot/Motor1 Torque Control Init Frame/SDO Set 0x6040:6 Frame/If Action Subsystem2 ==
  In1 : Inport
  Action Port : ActionPort  ActionPortLabel=else
  Out1 : Outport
  wires:
  In1/1 -> Out1/1

== system Robot/Motor1 Torque Control Init Frame/SDO Set 0x6040:6 Frame/If Action Subsystem3 ==
  In1 : Inport
  Action Port : ActionPort  ActionPortLabel=if((u1 == u2))
  Discrete-Time Integrator : DiscreteIntegrator  SampleTime=-1  ICPrevOutput=DiscIntNeverNeededParam  ICPrevScaledInput=DiscIntNeverNeededParam
  Out1 : Outport
  wires:
  In1/1 -> Discrete-Time Integrator/1
  Discrete-Time Integrator/1 -> Out1/1

== system Robot/Motor1 Torque Control Init Frame/SDO Set 0x6040:6 Frame/If Action Subsystem5 ==
  In1 : Inport
  Action Port : ActionPort  ActionPortLabel=if((u1 == 2))
  Out1 : Outport
  wires:
  In1/1 -> Out1/1

== system Robot/Motor1 Torque Control Init Frame/SDO Set 0x6040:6 Frame/If Action Subsystem6 ==
  In1 : Inport
  Action Port : ActionPort  ActionPortLabel=else
  Out1 : Outport
  wires:
  In1/1 -> Out1/1

== system Robot/Motor1 Torque Control Init Frame/SDO Set 0x6040:6 Frame/If Action Subsystem7 ==
  In1 : Inport
  Action Port : ActionPort  ActionPortLabel=if((u1 == 4663))
  Discrete-Time Integrator : DiscreteIntegrator  SampleTime=-1  ICPrevOutput=DiscIntNeverNeededParam  ICPrevScaledInput=DiscIntNeverNeededParam
  Out1 : Outport
  wires:
  In1/1 -> Discrete-Time Integrator/1
  Discrete-Time Integrator/1 -> Out1/1

== system Robot/Motor1 Torque Control Init Frame/SDO Set 0x6040:7 Frame/If Action Subsystem1 ==
  In1 : Inport
  Action Port : ActionPort  ActionPortLabel=if((u1 >= 0.1))
  Out1 : Outport
  wires:
  In1/1 -> Out1/1

== system Robot/Motor1 Torque Control Init Frame/SDO Set 0x6040:7 Frame/If Action Subsystem2 ==
  In1 : Inport
  Action Port : ActionPort  ActionPortLabel=else
  Out1 : Outport
  wires:
  In1/1 -> Out1/1

== system Robot/Motor1 Torque Control Init Frame/SDO Set 0x6040:7 Frame/If Action Subsystem3 ==
  In1 : Inport
  Action Port : ActionPort  ActionPortLabel=if((u1 == u2))
  Discrete-Time Integrator : DiscreteIntegrator  SampleTime=-1  ICPrevOutput=DiscIntNeverNeededParam  ICPrevScaledInput=DiscIntNeverNeededParam
  Out1 : Outport
  wires:
  In1/1 -> Discrete-Time Integrator/1
  Discrete-Time Integrator/1 -> Out1/1

== system Robot/Motor1 Torque Control Init Frame/SDO Set 0x6040:7 Frame/If Action Subsystem5 ==
  In1 : Inport
  Action Port : ActionPort  ActionPortLabel=if((u1 == 2))
  Out1 : Outport
  wires:
  In1/1 -> Out1/1

== system Robot/Motor1 Torque Control Init Frame/SDO Set 0x6040:7 Frame/If Action Subsystem6 ==
  In1 : Inport
  Action Port : ActionPort  ActionPortLabel=else
  Out1 : Outport
  wires:
  In1/1 -> Out1/1

== system Robot/Motor1 Torque Control Init Frame/SDO Set 0x6040:7 Frame/If Action Subsystem7 ==
  In1 : Inport
  Action Port : ActionPort  ActionPortLabel=if((u1 == 4663))
  Discrete-Time Integrator : DiscreteIntegrator  SampleTime=-1  ICPrevOutput=DiscIntNeverNeededParam  ICPrevScaledInput=DiscIntNeverNeededParam
  Out1 : Outport
  wires:
  In1/1 -> Discrete-Time Integrator/1
  Discrete-Time Integrator/1 -> Out1/1

== system Robot/Motor1 Torque Control Init Frame/SDO Set 0x6060:10 Frame/If Action Subsystem5 ==
  In1 : Inport
  Action Port : ActionPort  ActionPortLabel=if((u1 == 2))
  Out1 : Outport
  wires:
  In1/1 -> Out1/1

== system Robot/Motor1 Torque Control Init Frame/SDO Set 0x6060:10 Frame/If Action Subsystem6 ==
  In1 : Inport
  Action Port : ActionPort  ActionPortLabel=else
  Out1 : Outport
  wires:
  In1/1 -> Out1/1

== system Robot/Motor1 Torque Control Init Frame/SDO Set 0x6060:10 Frame/If Action Subsystem7 ==
  In1 : Inport
  Action Port : ActionPort  ActionPortLabel=if((u1 == 4663))
  Discrete-Time Integrator : DiscreteIntegrator  SampleTime=-1  ICPrevOutput=DiscIntNeverNeededParam  ICPrevScaledInput=DiscIntNeverNeededParam
  Out1 : Outport
  wires:
  In1/1 -> Discrete-Time Integrator/1
  Discrete-Time Integrator/1 -> Out1/1

== system Robot/Motor1 Torque Control Init Frame/SDO Set 0x6060:6 Frame/If Action Subsystem5 ==
  In1 : Inport
  Action Port : ActionPort  ActionPortLabel=if((u1 == 2))
  Out1 : Outport
  wires:
  In1/1 -> Out1/1

== system Robot/Motor1 Torque Control Init Frame/SDO Set 0x6060:6 Frame/If Action Subsystem6 ==
  In1 : Inport
  Action Port : ActionPort  ActionPortLabel=else
  Out1 : Outport
  wires:
  In1/1 -> Out1/1

== system Robot/Motor1 Torque Control Init Frame/SDO Set 0x6060:6 Frame/If Action Subsystem7 ==
  In1 : Inport
  Action Port : ActionPort  ActionPortLabel=if((u1 == 4663))
  Discrete-Time Integrator : DiscreteIntegrator  SampleTime=-1  ICPrevOutput=DiscIntNeverNeededParam  ICPrevScaledInput=DiscIntNeverNeededParam
  Out1 : Outport
  wires:
  In1/1 -> Discrete-Time Integrator/1
  Discrete-Time Integrator/1 -> Out1/1

== system Robot/Motor1 Torque Control Init Frame/SDO Set 0x6080:-1 Frame/If Action Subsystem5 ==
  In1 : Inport
  Action Port : ActionPort  ActionPortLabel=if((u1 == 2))
  Out1 : Outport
  wires:
  In1/1 -> Out1/1

== system Robot/Motor1 Torque Control Init Frame/SDO Set 0x6080:-1 Frame/If Action Subsystem6 ==
  In1 : Inport
  Action Port : ActionPort  ActionPortLabel=else
  Out1 : Outport
  wires:
  In1/1 -> Out1/1

== system Robot/Motor1 Torque Control Init Frame/SDO Set 0x6080:-1 Frame/If Action Subsystem7 ==
  In1 : Inport
  Action Port : ActionPort  ActionPortLabel=if((u1 == 4663))
  Discrete-Time Integrator : DiscreteIntegrator  SampleTime=-1  ICPrevOutput=DiscIntNeverNeededParam  ICPrevScaledInput=DiscIntNeverNeededParam
  Out1 : Outport
  wires:
  In1/1 -> Discrete-Time Integrator/1
  Discrete-Time Integrator/1 -> Out1/1

== system Robot/Motor1 Torque Control Init Frame/SDO Set 0x6098:35 Frame/If Action Subsystem5 ==
  In1 : Inport
  Action Port : ActionPort  ActionPortLabel=if((u1 == 2))
  Out1 : Outport
  wires:
  In1/1 -> Out1/1

== system Robot/Motor1 Torque Control Init Frame/SDO Set 0x6098:35 Frame/If Action Subsystem6 ==
  In1 : Inport
  Action Port : ActionPort  ActionPortLabel=else
  Out1 : Outport
  wires:
  In1/1 -> Out1/1

== system Robot/Motor1 Torque Control Init Frame/SDO Set 0x6098:35 Frame/If Action Subsystem7 ==
  In1 : Inport
  Action Port : ActionPort  ActionPortLabel=if((u1 == 4663))
  Discrete-Time Integrator : DiscreteIntegrator  SampleTime=-1  ICPrevOutput=DiscIntNeverNeededParam  ICPrevScaledInput=DiscIntNeverNeededParam
  Out1 : Outport
  wires:
  In1/1 -> Discrete-Time Integrator/1
  Discrete-Time Integrator/1 -> Out1/1

== system Robot/Motor1 Torque Control Init Frame/Set MasterState to OP Frame/If Action Subsystem5 ==
  In1 : Inport
  Action Port : ActionPort  ActionPortLabel=if((u1 > 0.1))
  Out1 : Outport
  wires:
  In1/1 -> Out1/1

== system Robot/Motor1 Torque Control Init Frame/Set MasterState to OP Frame/If Action Subsystem6 ==
  In1 : Inport
  Action Port : ActionPort  ActionPortLabel=else
  Out1 : Outport
  wires:
  In1/1 -> Out1/1
